simulink model "PthSet_TrqCalc"  (R2016b)
settings: configuration reference "CodeGenConfigSet" (kept outside this file)
values from neighbouring files (symbols this model uses):
  PthSet_dtrqRmpDwn_CUR = Calibration.Parameter    [init_PthSet_TrqCalc.m]    (also in init_PthSet_TrqCalc_SIL.m = Simulink.Parameter)
  PthSet_dtrqRmpDwn_CURX = Calibration.Parameter    [init_PthSet_TrqCalc.m]    (also in init_PthSet_TrqCalc_SIL.m = Simulink.Parameter)
  PthSet_dtrqRmpDwnDfl_C = Calibration.Parameter    [init_PthSet_TrqCalc.m]    (also in init_PthSet_TrqCalc_SIL.m = Simulink.Parameter)
  PthSet_tiRmpStrt_CUR = Calibration.Parameter    [init_PthSet_TrqCalc.m]    (also in init_PthSet_TrqCalc_SIL.m = Simulink.Parameter)
  PthSet_tiRmpStrt_CURX = Calibration.Parameter    [init_PthSet_TrqCalc.m]    (also in init_PthSet_TrqCalc_SIL.m = Simulink.Parameter)
  PthSet_tiRmpStrtDfl_C = Calibration.Parameter    [init_PthSet_TrqCalc.m]    (also in init_PthSet_TrqCalc_SIL.m = Simulink.Parameter)
  PthSet_tiSwtOff_CUR = Calibration.Parameter    [init_PthSet_TrqCalc.m]    (also in init_PthSet_TrqCalc_SIL.m = Simulink.Parameter)
  PthSet_tiSwtOff_CURX = Calibration.Parameter    [init_PthSet_TrqCalc.m]    (also in init_PthSet_TrqCalc_SIL.m = Simulink.Parameter)
  PthSet_tiSwtOffDfl_C = Calibration.Parameter    [init_PthSet_TrqCalc.m]    (also in init_PthSet_TrqCalc_SIL.m = Simulink.Parameter)
  PthSet_trqOffs_C = Calibration.Parameter    [init_PthSet_TrqCalc.m]    (also in init_PthSet_TrqCalc_SIL.m = Simulink.Parameter)
  TRQ_ZERO = fi(0,Trq_Nm)    [init_PthSet_TrqCalc.m]    (also in init_PthSet_TrqCalc_SIL.m)
undefined symbols (not defined in the file or in its folder): EngState_conv, HPUn_etaPmp_MAPY, PthSet_TrqCalc_DT
libraries: simulink x4, CXLib x4
settings Model: Creator=Wollf  LastModifiedBy=xuxingpei
settings ConfigSetRef: SourceLocation=Base Workspace

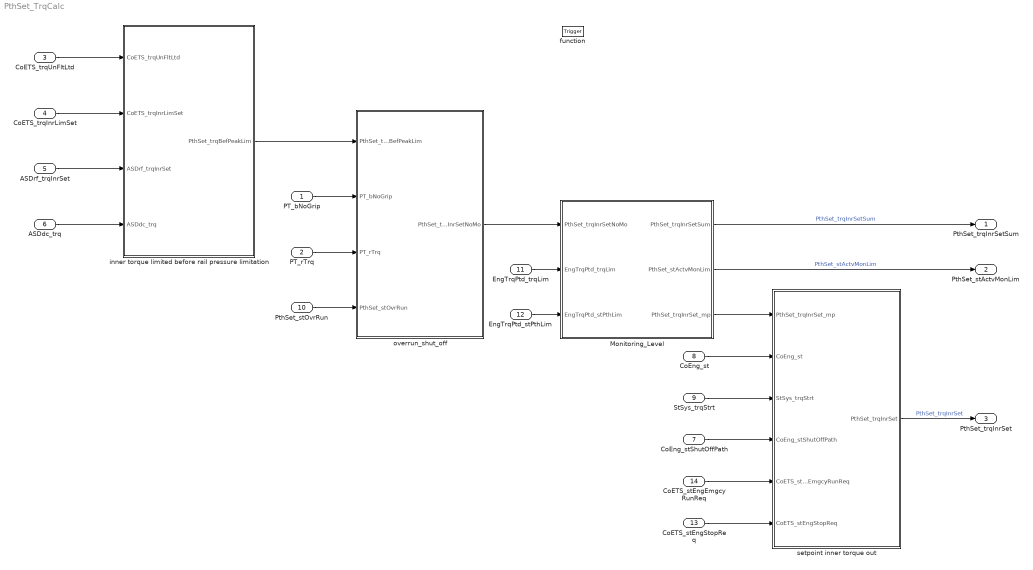
== system PthSet_TrqCalc ==
  PT_bNoGrip : Inport  Description=Grip reliable exclude  OutMin=0  OutMax=1  OutDataTypeStr=boolean
  PT_rTrq : Inport  Description=Powertrain torque ratio  Port=2  OutMin=-100  OutMax=100  OutDataTypeStr=TransRatio
  CoETS_trqUnFltLtd : Inport  Tag=Nm  Description=Limited idle speed governor torque  Port=3  OutMin=-3276  OutMax=3276  OutDataTypeStr=Trq_Nm
  CoETS_trqInrLimSet : Inport  Tag=Nm  Description=Limitation torque without the part of the speed governor  Port=4  OutMin=-3000  OutMax=3000  OutDataTypeStr=Trq_Nm
  ASDrf_trqInrSet : Inport  Tag=Nm  Description=ASD reference filter torque output  Port=5  OutMin=-3000  OutMax=3000  OutDataTypeStr=Trq_Nm
  ASDdc_trq : Inport  Tag=Nm  Description=ASD disturbance compensator torque output  Port=6  OutMin=-3000  OutMax=3000  OutDataTypeStr=Trq_Nm
  CoEng_stShutOffPath : Inport  Description=Active shut-off paths resulting from active reversible,irreversible and afterrun shut-off paths  Port=7  OutMin=0  OutMax=65535  OutDataTypeStr=State_uint16
  CoEng_st : Inport  Description=Engine coordinator state  Port=8  OutDataTypeStr=Enum: EngState_conv
  StSys_trqStrt : Inport  Tag=Nm  Description=Engine starting torque  Port=9  OutMin=-3000  OutMax=3000  OutDataTypeStr=Trq_Nm
  PthSet_stOvrRun : Inport  Description=State of overrun detection (0: No overrun; 1: overrun)  Port=10  OutMin=0  OutMax=1  OutDataTypeStr=boolean
  EngTrqPtd_trqLim : Inport  Tag=Nm  Description=Set path torque limitation from ECU monitoring  Port=11  OutMin=-3276  OutMax=3276  OutDataTypeStr=Trq_Nm
  EngTrqPtd_stPthLim : Inport  Description=State of engine torque limitation from ECU monitoring  Port=12  OutMin=0  OutMax=255  OutDataTypeStr=State_uint8
  CoETS_stEngStopReq : Inport  Description=Tbox Engine stop request  Port=13  OutMin=0  OutMax=1  OutDataTypeStr=boolean
  CoETS_stEngEmgcyRunReq : Inport  Description=Tbox Engine emergency start request  Port=14  OutMin=0  OutMax=1  OutDataTypeStr=boolean
  function : TriggerPort  TriggerType=function-call  VariantControl=Variant
  Monitoring_Level : Subsystem
  inner torque limited before rail pressure limitation : Subsystem
  overrun_shut_off : Subsystem
  setpoint inner torque out : Subsystem
  PthSet_trqInrSetSum : Outport  Tag=Nm  Description=Sum of inner set torque  OutMin=-3000  OutMax=3276.7  OutDataTypeStr=Trq_Nm
  PthSet_stActvMonLim : Outport  Description=State of monitoring limitation  Port=2  OutMin=0  OutMax=255  OutDataTypeStr=State_uint8
  PthSet_trqInrSet : Outport  Tag=Nm  Description=Inner torque set value after monitoring limitation  Port=3  OutMin=-3000  OutMax=3276.7  OutDataTypeStr=Trq_Nm
  wires:
  PT_bNoGrip/1 -> overrun_shut_off/2(PT_bNoGrip)
  PT_rTrq/1 -> overrun_shut_off/3(PT_rTrq)
  Monitoring_Level/2(PthSet_stActvMonLim) -> PthSet_stActvMonLim/1  "PthSet_stActvMonLim"
  Monitoring_Level/1(PthSet_trqInrSetSum) -> PthSet_trqInrSetSum/1  "PthSet_trqInrSetSum"
  PthSet_stOvrRun/1 -> overrun_shut_off/4(PthSet_stOvrRun)
  overrun_shut_off/1(PthSet_trqInrSetNoMo) -> Monitoring_Level/1(PthSet_trqInrSetNoMo)
  CoETS_trqUnFltLtd/1 -> inner torque limited before rail pressure limitation/1(CoETS_trqUnFltLtd)
  CoETS_trqInrLimSet/1 -> inner torque limited before rail pressure limitation/2(CoETS_trqInrLimSet)
  ASDrf_trqInrSet/1 -> inner torque limited before rail pressure limitation/3(ASDrf_trqInrSet)
  ASDdc_trq/1 -> inner torque limited before rail pressure limitation/4(ASDdc_trq)
  CoEng_st/1 -> setpoint inner torque out/2(CoEng_st)
  StSys_trqStrt/1 -> setpoint inner torque out/3(StSys_trqStrt)
  Monitoring_Level/3(PthSet_trqInrSet_mp) -> setpoint inner torque out/1(PthSet_trqInrSet_mp)
  setpoint inner torque out/1(PthSet_trqInrSet) -> PthSet_trqInrSet/1  "PthSet_trqInrSet"
  inner torque limited before rail pressure limitation/1(PthSet_trqBefPeakLim) -> overrun_shut_off/1(PthSet_trqBefPeakLim)
  CoEng_stShutOffPath/1 -> setpoint inner torque out/4(CoEng_stShutOffPath)
  EngTrqPtd_trqLim/1 -> Monitoring_Level/2(EngTrqPtd_trqLim)
  EngTrqPtd_stPthLim/1 -> Monitoring_Level/3(EngTrqPtd_stPthLim)
  CoETS_stEngEmgcyRunReq/1 -> setpoint inner torque out/5(CoETS_stEngEmgcyRunReq)
  CoETS_stEngStopReq/1 -> setpoint inner torque out/6(CoETS_stEngStopReq)

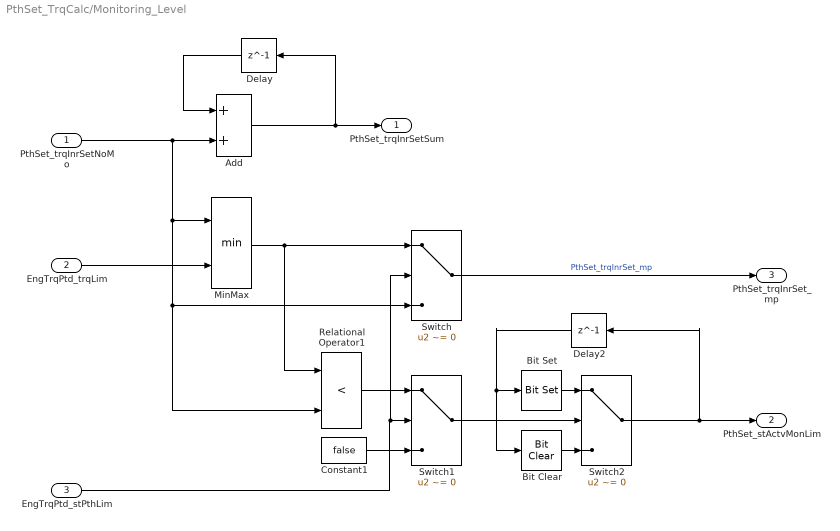
== system PthSet_TrqCalc/Monitoring_Level ==
  PthSet_trqInrSetNoMo : Inport
  EngTrqPtd_trqLim : Inport  Port=2
  EngTrqPtd_stPthLim : Inport  Port=3
  Add : Sum  SaturateOnIntegerOverflow=on  InputSameDT=on
  Bit Clear : simulink/Logic and Bit Operations/Bit Clear  iBit=0
  Bit Set : simulink/Logic and Bit Operations/Bit Set  iBit=0
  Constant1 : Constant  Value=false  OutDataTypeStr=Inherit: Inherit via back propagation
  Delay : Delay  DelayLength=1  InitialCondition=0
  Delay2 : Delay  DelayLength=1  InitialCondition=0
  MinMax : MinMax  Inputs=2  InputSameDT=on
  Relational Operator1 : RelationalOperator  Operator=<  OutDataTypeStr=boolean  RndMeth=Simplest  InputSameDT=on
  Switch : Switch  Criteria=u2 ~= 0  InputSameDT=on
  Switch1 : Switch  Criteria=u2 ~= 0  InputSameDT=on
  Switch2 : Switch  Criteria=u2 ~= 0  InputSameDT=on
  PthSet_trqInrSetSum : Outport
  PthSet_stActvMonLim : Outport  Port=2
  PthSet_trqInrSet_mp : Outport  Port=3
  wires:
  Delay2/1 -> Bit Set/1, Bit Clear/1
  Bit Clear/1 -> Switch2/3
  Bit Set/1 -> Switch2/1
  Switch2/1 -> PthSet_stActvMonLim/1, Delay2/1
  Switch1/1 -> Switch2/2
  Switch/1 -> PthSet_trqInrSet_mp/1  "PthSet_trqInrSet_mp"
  EngTrqPtd_stPthLim/1 -> Switch1/2, Switch/2
  Constant1/1 -> Switch1/3
  Relational Operator1/1 -> Switch1/1
  MinMax/1 -> Switch/1, Relational Operator1/1
  EngTrqPtd_trqLim/1 -> MinMax/2
  Delay/1 -> Add/1
  Add/1 -> PthSet_trqInrSetSum/1, Delay/1
  PthSet_trqInrSetNoMo/1 -> Add/2, MinMax/1, Switch/3, Relational Operator1/2

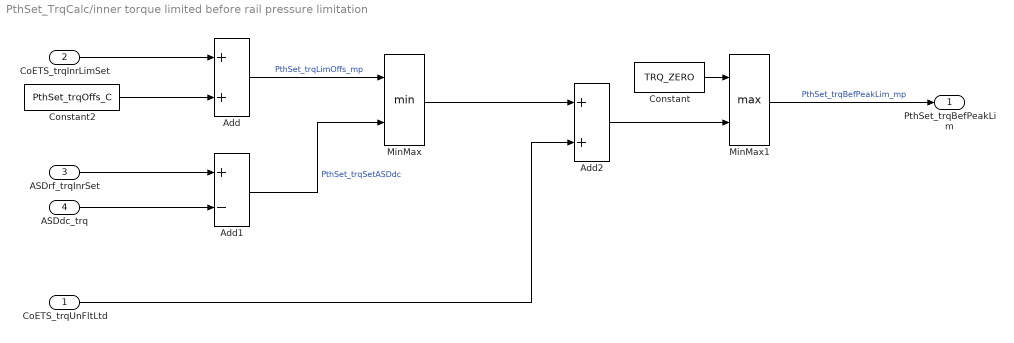
== system PthSet_TrqCalc/inner torque limited before rail pressure limitation ==
  CoETS_trqUnFltLtd : Inport
  CoETS_trqInrLimSet : Inport  Port=2
  ASDrf_trqInrSet : Inport  Port=3
  ASDdc_trq : Inport  Port=4
  Add : Sum  SaturateOnIntegerOverflow=on  InputSameDT=on
  Add1 : Sum  Inputs=+-  OutDataTypeStr=Inherit: Inherit via back propagation  SaturateOnIntegerOverflow=on  InputSameDT=on
  Add2 : Sum  SaturateOnIntegerOverflow=on  InputSameDT=on
  Constant : Constant  Value=TRQ_ZERO  OutDataTypeStr=Inherit: Inherit via back propagation
  Constant2 : Constant  Value=PthSet_trqOffs_C
  MinMax : MinMax  Inputs=2  InputSameDT=on
  MinMax1 : MinMax  Function=max  Inputs=2  InputSameDT=on
  PthSet_trqBefPeakLim : Outport
  wires:
  Constant2/1 -> Add/2
  ASDdc_trq/1 -> Add1/2
  Add2/1 -> MinMax1/2
  CoETS_trqInrLimSet/1 -> Add/1
  ASDrf_trqInrSet/1 -> Add1/1
  Add1/1 -> MinMax/2  "PthSet_trqSetASDdc"
  Add/1 -> MinMax/1  "PthSet_trqLimOffs_mp"
  CoETS_trqUnFltLtd/1 -> Add2/2
  MinMax/1 -> Add2/1
  Constant/1 -> MinMax1/1
  MinMax1/1 -> PthSet_trqBefPeakLim/1  "PthSet_trqBefPeakLim_mp"

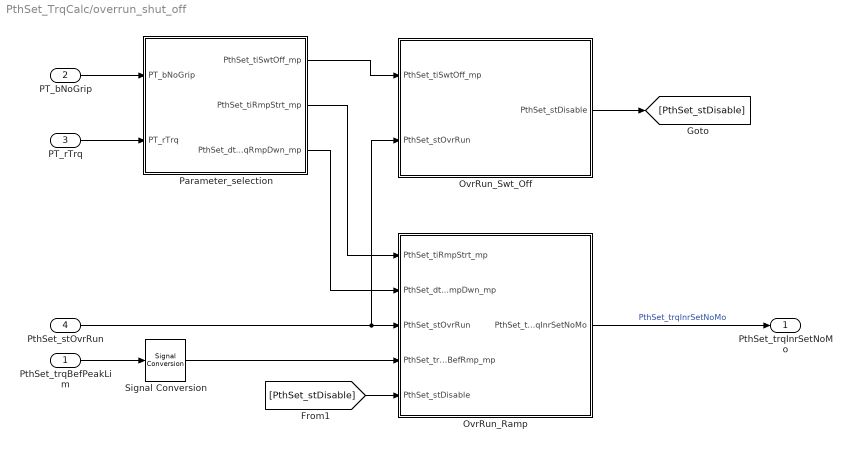
== system PthSet_TrqCalc/overrun_shut_off ==
  PthSet_trqBefPeakLim : Inport
  PT_bNoGrip : Inport  Port=2
  PT_rTrq : Inport  Port=3
  PthSet_stOvrRun : Inport  Port=4
  OvrRun_Ramp : Subsystem
  OvrRun_Swt_Off : Subsystem
  Parameter_selection : Subsystem
  Signal Conversion : SignalConversion  OverrideOpt=off
  PthSet_trqInrSetNoMo : Outport
  wires:
  PthSet_stOvrRun/1 -> OvrRun_Swt_Off/2(PthSet_stOvrRun), OvrRun_Ramp/3(PthSet_stOvrRun)
  Parameter_selection/2(PthSet_tiRmpStrt_mp) -> OvrRun_Ramp/1(PthSet_tiRmpStrt_mp)
  Parameter_selection/3(PthSet_dtrqRmpDwn_mp) -> OvrRun_Ramp/2(PthSet_dtrqRmpDwn_mp)
  Parameter_selection/1("PthSet_tiSwtOff_mp ") -> OvrRun_Swt_Off/1(PthSet_tiSwtOff_mp)
  OvrRun_Swt_Off/1(PthSet_stDisable) -> [PthSet_stDisable]
  PthSet_trqBefPeakLim/1 -> Signal Conversion/1
  PT_rTrq/1 -> Parameter_selection/2(PT_rTrq)
  PT_bNoGrip/1 -> Parameter_selection/1(PT_bNoGrip)
  [PthSet_stDisable] -> OvrRun_Ramp/5(PthSet_stDisable)
  OvrRun_Ramp/1(PthSet_trqInrSetNoMo) -> PthSet_trqInrSetNoMo/1  "PthSet_trqInrSetNoMo"
  Signal Conversion/1 -> OvrRun_Ramp/4(PthSet_trqBefRmp_mp)

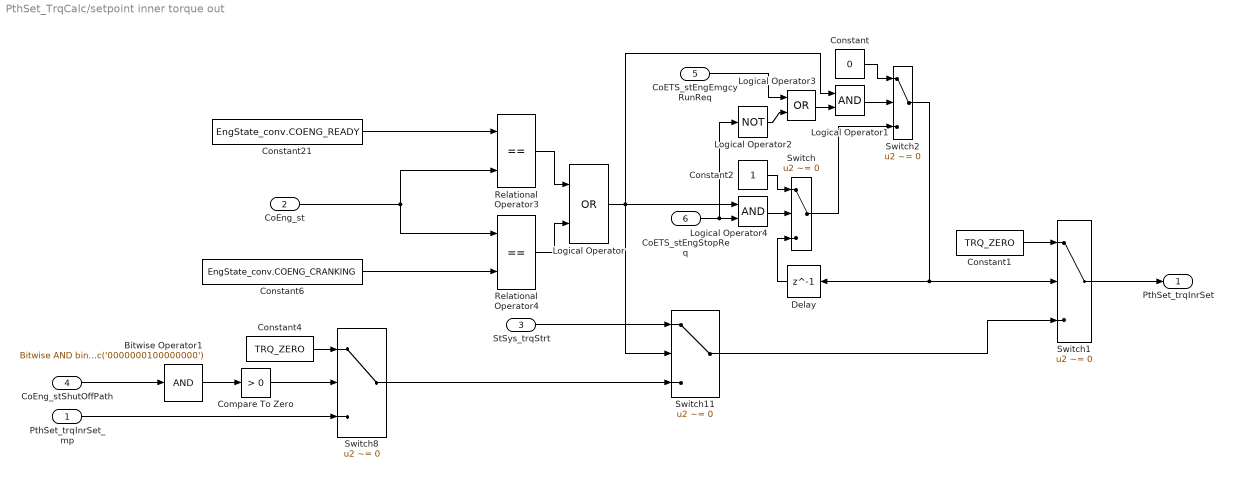
== system PthSet_TrqCalc/setpoint inner torque out ==
  PthSet_trqInrSet_mp : Inport
  CoEng_st : Inport  Port=2
  StSys_trqStrt : Inport  Port=3
  CoEng_stShutOffPath : Inport  Port=4
  CoETS_stEngEmgcyRunReq : Inport  Port=5
  CoETS_stEngStopReq : Inport  Port=6
  Bitwise Operator1 : simulink/Logic and Bit Operations/Bitwise Operator  logicop=AND  UseBitMask=on  BitMask=bin2dec('0000000100000000')  BitMaskRealWorld=Stored Integer
  Compare To Zero : simulink/Logic and Bit Operations/Compare To Zero  relop=>  OutDataTypeStr=boolean
  Constant : Constant  Value=0  OutDataTypeStr=Inherit: Inherit via back propagation
  Constant1 : Constant  Value=TRQ_ZERO  OutDataTypeStr=Inherit: Inherit via back propagation
  Constant2 : Constant  OutDataTypeStr=Inherit: Inherit via back propagation
  Constant21 : Constant  Value=EngState_conv.COENG_READY  OutDataTypeStr=Inherit: Inherit via back propagation
  Constant4 : Constant  Value=TRQ_ZERO  OutDataTypeStr=Inherit: Inherit via back propagation
  Constant6 : Constant  Value=EngState_conv.COENG_CRANKING  OutDataTypeStr=Inherit: Inherit via back propagation
  Delay : Delay  DelayLength=1  InitialCondition=0
  Logical Operator : Logic  Operator=OR  OutDataTypeStr=boolean
  Logical Operator1 : Logic  AllPortsSameDT=off  OutDataTypeStr=boolean
  Logical Operator2 : Logic  Operator=NOT  AllPortsSameDT=off  OutDataTypeStr=boolean
  Logical Operator3 : Logic  Operator=OR  AllPortsSameDT=off  OutDataTypeStr=boolean
  Logical Operator4 : Logic  AllPortsSameDT=off  OutDataTypeStr=boolean
  Relational Operator3 : RelationalOperator  Operator===  OutDataTypeStr=boolean  RndMeth=Simplest  InputSameDT=on
  Relational Operator4 : RelationalOperator  Operator===  OutDataTypeStr=boolean  RndMeth=Simplest  InputSameDT=on
  Switch : Switch  Criteria=u2 ~= 0
  Switch1 : Switch  Criteria=u2 ~= 0  InputSameDT=on
  Switch11 : Switch  Criteria=u2 ~= 0  InputSameDT=on
  Switch2 : Switch  Criteria=u2 ~= 0
  Switch8 : Switch  Criteria=u2 ~= 0  InputSameDT=on
  PthSet_trqInrSet : Outport
  wires:
  Switch8/1 -> Switch11/3
  CoEng_st/1 -> Relational Operator3/2, Relational Operator4/1
  CoEng_stShutOffPath/1 -> Bitwise Operator1/1
  StSys_trqStrt/1 -> Switch11/1
  Constant6/1 -> Relational Operator4/2
  Constant21/1 -> Relational Operator3/1
  Constant4/1 -> Switch8/1
  Logical Operator/1 -> Logical Operator1/1, Logical Operator4/1, Switch11/2
  Relational Operator3/1 -> Logical Operator/1
  Relational Operator4/1 -> Logical Operator/2
  PthSet_trqInrSet_mp/1 -> Switch8/3
  Bitwise Operator1/1 -> Compare To Zero/1
  Compare To Zero/1 -> Switch8/2
  Switch11/1 -> Switch1/3
  Switch1/1 -> PthSet_trqInrSet/1
  Constant1/1 -> Switch1/1
  Switch2/1 -> Delay/1, Switch1/2
  Switch/1 -> Switch2/3
  Constant/1 -> Switch2/1
  Constant2/1 -> Switch/1
  Logical Operator1/1 -> Switch2/2
  Logical Operator2/1 -> Logical Operator3/2
  Logical Operator3/1 -> Logical Operator1/2
  CoETS_stEngEmgcyRunReq/1 -> Logical Operator3/1
  Logical Operator4/1 -> Switch/2
  CoETS_stEngStopReq/1 -> Logical Operator2/1, Logical Operator4/2
  Delay/1 -> Switch/3

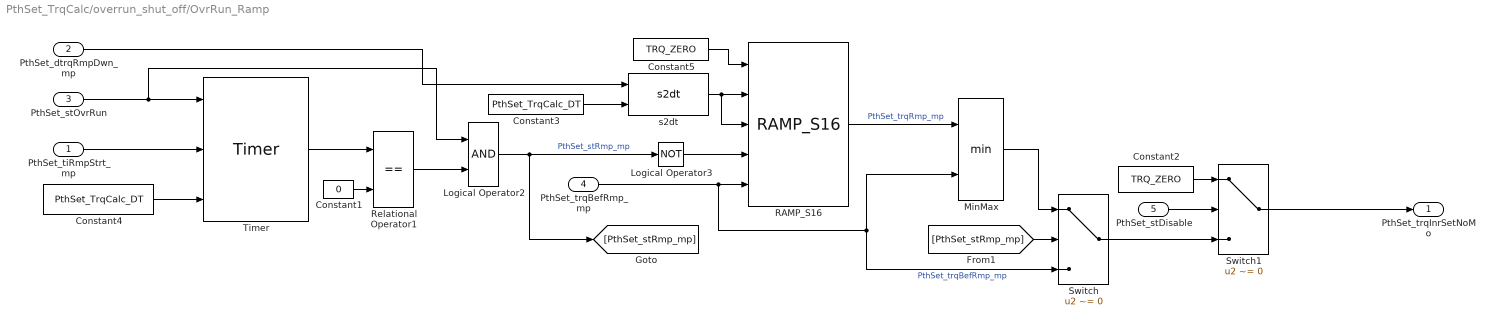
== system PthSet_TrqCalc/overrun_shut_off/OvrRun_Ramp ==
  PthSet_tiRmpStrt_mp : Inport
  PthSet_dtrqRmpDwn_mp : Inport  Port=2
  PthSet_stOvrRun : Inport  Port=3
  PthSet_trqBefRmp_mp : Inport  Port=4
  PthSet_stDisable : Inport  Port=5
  Constant1 : Constant  Value=0  OutDataTypeStr=Inherit: Inherit via back propagation
  Constant2 : Constant  Value=TRQ_ZERO  OutDataTypeStr=Inherit: Inherit via back propagation
  Constant3 : Constant  Value=PthSet_TrqCalc_DT  OutDataTypeStr=Inherit: Inherit via back propagation
  Constant4 : Constant  Value=PthSet_TrqCalc_DT  OutDataTypeStr=Inherit: Inherit via back propagation
  Constant5 : Constant  Value=TRQ_ZERO  OutDataTypeStr=Inherit: Inherit via back propagation
  Logical Operator2 : Logic  AllPortsSameDT=off  OutDataTypeStr=boolean
  Logical Operator3 : Logic  Operator=NOT  AllPortsSameDT=off  OutDataTypeStr=boolean
  MinMax : MinMax  Inputs=2  InputSameDT=on
  RAMP_S16 : CXLib/RAMP_S16
  Relational Operator1 : RelationalOperator  Operator===  OutDataTypeStr=boolean  RndMeth=Simplest  InputSameDT=on
  Switch : Switch  Criteria=u2 ~= 0  InputSameDT=on
  Switch1 : Switch  Criteria=u2 ~= 0  InputSameDT=on
  Timer : CXLib/Timer
  s2dt : CXLib/s2dt
  PthSet_trqInrSetNoMo : Outport
  wires:
  Logical Operator3/1 -> RAMP_S16/4
  Relational Operator1/1 -> Logical Operator2/2
  PthSet_trqBefRmp_mp/1 -> Switch/3, MinMax/2, RAMP_S16/5  "PthSet_trqBefRmp_mp"
  Logical Operator2/1 -> [PthSet_stRmp_mp], Logical Operator3/1  "PthSet_stRmp_mp"
  RAMP_S16/1 -> MinMax/1  "PthSet_trqRmp_mp"
  Constant1/1 -> Relational Operator1/2
  Timer/1 -> Relational Operator1/1
  Constant5/1 -> RAMP_S16/1
  s2dt/1 -> RAMP_S16/2, RAMP_S16/3
  PthSet_tiRmpStrt_mp/1 -> Timer/2
  PthSet_stOvrRun/1 -> Timer/1, Logical Operator2/1
  Constant2/1 -> Switch1/1
  Switch/1 -> Switch1/3
  Switch1/1 -> PthSet_trqInrSetNoMo/1
  MinMax/1 -> Switch/1
  PthSet_stDisable/1 -> Switch1/2
  [PthSet_stRmp_mp] -> Switch/2
  Constant4/1 -> Timer/3
  PthSet_dtrqRmpDwn_mp/1 -> s2dt/1
  Constant3/1 -> s2dt/2

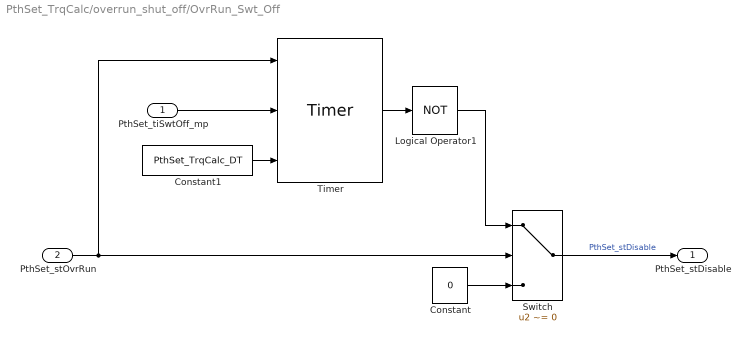
== system PthSet_TrqCalc/overrun_shut_off/OvrRun_Swt_Off ==
  PthSet_tiSwtOff_mp : Inport
  PthSet_stOvrRun : Inport  Port=2
  Constant : Constant  Value=0  OutDataTypeStr=Inherit: Inherit via back propagation
  Constant1 : Constant  Value=PthSet_TrqCalc_DT  OutDataTypeStr=Inherit: Inherit via back propagation
  Logical Operator1 : Logic  Operator=NOT  AllPortsSameDT=off  OutDataTypeStr=boolean
  Switch : Switch  Criteria=u2 ~= 0  InputSameDT=on
  Timer : CXLib/Timer
  PthSet_stDisable : Outport
  wires:
  Switch/1 -> PthSet_stDisable/1  "PthSet_stDisable"
  Logical Operator1/1 -> Switch/1
  Timer/1 -> Logical Operator1/1
  PthSet_tiSwtOff_mp/1 -> Timer/2
  Constant/1 -> Switch/3
  PthSet_stOvrRun/1 -> Timer/1, Switch/2
  Constant1/1 -> Timer/3

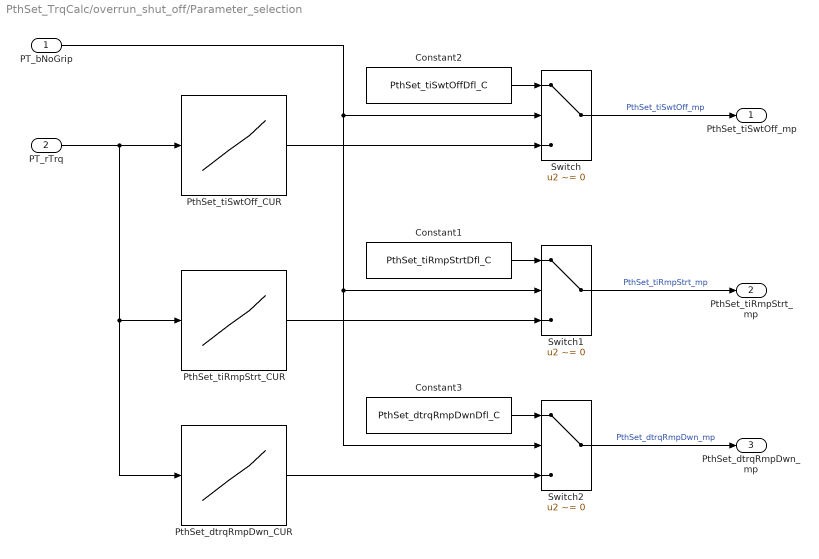
== system PthSet_TrqCalc/overrun_shut_off/Parameter_selection ==
  PT_bNoGrip : Inport
  PT_rTrq : Inport  Port=2
  Constant1 : Constant  Value=PthSet_tiRmpStrtDfl_C
  Constant2 : Constant  Value=PthSet_tiSwtOffDfl_C
  Constant3 : Constant  Value=PthSet_dtrqRmpDwnDfl_C
  PthSet_dtrqRmpDwn_CUR : Lookup_n-D  NumberOfTableDimensions=1  BreakpointsForDimension1=PthSet_dtrqRmpDwn_CURX  BreakpointsForDimension2=HPUn_etaPmp_MAPY  IndexSearchMethod=Linear search  BeginIndexSearchUsingPreviousIndexResult=on  Table=PthSet_dtrqRmpDwn_CUR  ExtrapMethod=Clip  UseLastTableValue=on  InternalRulePriority=Speed  OutDataTypeStr=Inherit: Inherit via back propagation  SaturateOnIntegerOverflow=on
  PthSet_tiRmpStrt_CUR : Lookup_n-D  NumberOfTableDimensions=1  BreakpointsForDimension1=PthSet_tiRmpStrt_CURX  BreakpointsForDimension2=HPUn_etaPmp_MAPY  IndexSearchMethod=Linear search  BeginIndexSearchUsingPreviousIndexResult=on  Table=PthSet_tiRmpStrt_CUR  ExtrapMethod=Clip  UseLastTableValue=on  InternalRulePriority=Speed  OutDataTypeStr=Inherit: Inherit via back propagation  SaturateOnIntegerOverflow=on
  PthSet_tiSwtOff_CUR : Lookup_n-D  NumberOfTableDimensions=1  BreakpointsForDimension1=PthSet_tiSwtOff_CURX  BreakpointsForDimension2=HPUn_etaPmp_MAPY  IndexSearchMethod=Linear search  BeginIndexSearchUsingPreviousIndexResult=on  Table=PthSet_tiSwtOff_CUR  ExtrapMethod=Clip  UseLastTableValue=on  InternalRulePriority=Speed  OutDataTypeStr=Inherit: Inherit via back propagation  SaturateOnIntegerOverflow=on
  Switch : Switch  Criteria=u2 ~= 0  InputSameDT=on
  Switch1 : Switch  Criteria=u2 ~= 0  InputSameDT=on
  Switch2 : Switch  Criteria=u2 ~= 0  InputSameDT=on
  "PthSet_tiSwtOff_mp " : Outport
  PthSet_tiRmpStrt_mp : Outport  Port=2
  PthSet_dtrqRmpDwn_mp : Outport  Port=3
  wires:
  Constant3/1 -> Switch2/1
  Constant1/1 -> Switch1/1
  Constant2/1 -> Switch/1
  Switch2/1 -> PthSet_dtrqRmpDwn_mp/1  "PthSet_dtrqRmpDwn_mp"
  Switch1/1 -> PthSet_tiRmpStrt_mp/1  "PthSet_tiRmpStrt_mp"
  PT_bNoGrip/1 -> Switch2/2, Switch1/2, Switch/2
  PthSet_dtrqRmpDwn_CUR/1 -> Switch2/3
  PthSet_tiRmpStrt_CUR/1 -> Switch1/3
  Switch/1 -> "PthSet_tiSwtOff_mp "/1  "PthSet_tiSwtOff_mp"
  PthSet_tiSwtOff_CUR/1 -> Switch/3
  PT_rTrq/1 -> PthSet_tiSwtOff_CUR/1, PthSet_tiRmpStrt_CUR/1, PthSet_dtrqRmpDwn_CUR/1
